simulink model "GoertzelFunction"  (R2014a)
settings: Solver=ode45  StartTime=0.0  StopTime=1  RelTol=1e-3
undefined symbols (not defined in the file): i
libraries: dspsigops x14, dspsrcs4 x7
settings Model: Creator=Tanvir  LastModifiedBy=Tanvir

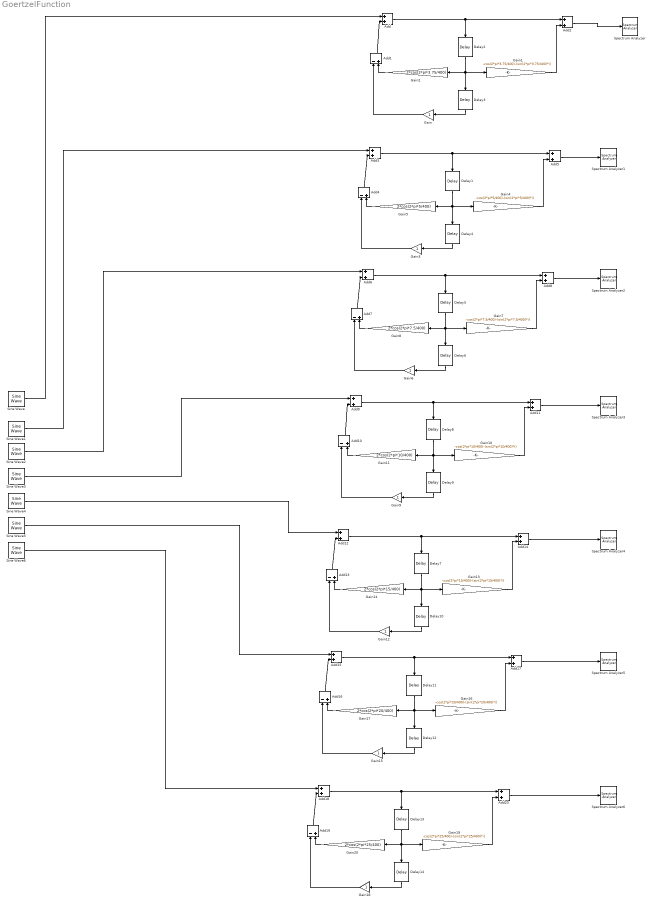
== system GoertzelFunction ==
  Add{,2..3,5..6,8..9,11..12,14..15,17..18,20} (14 alike) : Sum
  Add{1,4,7,10,13,16,19} (7 alike) : Sum  Inputs=-+
  Delay{1..14} (14 alike) : dspsigops/Delay  InputProcessing=Columns as channels (frame based)  dly_unit=Samples  delay=1  ic_detail=off  dif_ic_for_ch=off  dif_ic_for_dly=off  ic=0  reset_popup=None
  Gain{,3,6,9,12,15,18} (7 alike) : Gain
  Gain1 : Gain  Gain=-cos(2*pi*3.75/400)-(sin(2*pi*3.75/400)*i)
  Gain10 : Gain  Gain=-cos(2*pi*10/400)-(sin(2*pi*10/400)*i)
  Gain11 : Gain  Gain=2*cos(2*pi*10/400)
  Gain13 : Gain  Gain=-cos(2*pi*15/400)-(sin(2*pi*15/400)*i)
  Gain14 : Gain  Gain=2*cos(2*pi*15/400)
  Gain16 : Gain  Gain=-cos(2*pi*20/400)-(sin(2*pi*20/400)*i)
  Gain17 : Gain  Gain=2*cos(2*pi*20/400)
  Gain19 : Gain  Gain=-cos(2*pi*25/400)-(sin(2*pi*25/400)*i)
  Gain2 : Gain  Gain=2*cos(2*pi*3.75/400)
  Gain20 : Gain  Gain=2*cos(2*pi*25/400)
  Gain4 : Gain  Gain=-cos(2*pi*5/400)-(sin(2*pi*5/400)*i)
  Gain5 : Gain  Gain=2*cos(2*pi*5/400)
  Gain7 : Gain  Gain=-cos(2*pi*7.5/400)-(sin(2*pi*7.5/400)*i)
  Gain8 : Gain  Gain=2*cos(2*pi*7.5/400)
  Sine Wave : dspsrcs4/Sine Wave  Amplitude=1  Frequency=75  Phase=0  SampleMode=Discrete  OutComplex=Real  CompMethod=Trigonometric fcn  TableSize=Speed  SampleTime=1/8000  SamplesPerFrame=1  ResetState=Restart at time zero  dataType=double  wordLen=16  udDataType=sfix(16)  fracBitsMode=Best precision  numFracBits=15  OutDataTypeStr=double  LastOutDataTypeStr=double
  Sine Wave1 : dspsrcs4/Sine Wave  Amplitude=1  Frequency=100  Phase=0  SampleMode=Discrete  OutComplex=Real  CompMethod=Trigonometric fcn  TableSize=Speed  SampleTime=1/8000  SamplesPerFrame=1  ResetState=Restart at time zero  dataType=double  wordLen=16  udDataType=sfix(16)  fracBitsMode=Best precision  numFracBits=15  OutDataTypeStr=double  LastOutDataTypeStr=double
  Sine Wave2 : dspsrcs4/Sine Wave  Amplitude=1  Frequency=150  Phase=0  SampleMode=Discrete  OutComplex=Real  CompMethod=Trigonometric fcn  TableSize=Speed  SampleTime=1/8000  SamplesPerFrame=1  ResetState=Restart at time zero  dataType=double  wordLen=16  udDataType=sfix(16)  fracBitsMode=Best precision  numFracBits=15  OutDataTypeStr=double  LastOutDataTypeStr=double
  Sine Wave3 : dspsrcs4/Sine Wave  Amplitude=1  Frequency=200  Phase=0  SampleMode=Discrete  OutComplex=Real  CompMethod=Trigonometric fcn  TableSize=Speed  SampleTime=1/8000  SamplesPerFrame=1  ResetState=Restart at time zero  dataType=double  wordLen=16  udDataType=sfix(16)  fracBitsMode=Best precision  numFracBits=15  OutDataTypeStr=double  LastOutDataTypeStr=double
  Sine Wave4 : dspsrcs4/Sine Wave  Amplitude=1  Frequency=300  Phase=0  SampleMode=Discrete  OutComplex=Real  CompMethod=Trigonometric fcn  TableSize=Speed  SampleTime=1/8000  SamplesPerFrame=1  ResetState=Restart at time zero  dataType=double  wordLen=16  udDataType=sfix(16)  fracBitsMode=Best precision  numFracBits=15  OutDataTypeStr=double  LastOutDataTypeStr=double
  Sine Wave5 : dspsrcs4/Sine Wave  Amplitude=1  Frequency=400  Phase=0  SampleMode=Discrete  OutComplex=Real  CompMethod=Trigonometric fcn  TableSize=Speed  SampleTime=1/8000  SamplesPerFrame=1  ResetState=Restart at time zero  dataType=double  wordLen=16  udDataType=sfix(16)  fracBitsMode=Best precision  numFracBits=15  OutDataTypeStr=double  LastOutDataTypeStr=double
  Sine Wave6 : dspsrcs4/Sine Wave  Amplitude=1  Frequency=500  Phase=0  SampleMode=Discrete  OutComplex=Real  CompMethod=Trigonometric fcn  TableSize=Speed  SampleTime=1/8000  SamplesPerFrame=1  ResetState=Restart at time zero  dataType=double  wordLen=16  udDataType=sfix(16)  fracBitsMode=Best precision  numFracBits=15  OutDataTypeStr=double  LastOutDataTypeStr=double
  Spectrum Analyzer{,1..6} (7 alike) : SpectrumAnalyzer
  wires:
  Delay2/1 -> Gain1/1, Gain2/1, Delay3/1
  Delay3/1 -> Gain/1
  Add/1 -> Add2/1, Delay2/1
  Gain/1 -> Add1/1
  Add1/1 -> Add/2
  Gain1/1 -> Add2/2
  Gain2/1 -> Add1/2
  Sine Wave/1 -> Add/1
  Delay1/1 -> Gain4/1, Gain5/1, Delay4/1
  Delay4/1 -> Gain3/1
  Add3/1 -> Add5/1, Delay1/1
  Gain3/1 -> Add4/1
  Add4/1 -> Add3/2
  Gain4/1 -> Add5/2
  Gain5/1 -> Add4/2
  Sine Wave1/1 -> Add3/1
  Delay5/1 -> Gain7/1, Gain8/1, Delay6/1
  Delay6/1 -> Gain6/1
  Add6/1 -> Add8/1, Delay5/1
  Gain6/1 -> Add7/1
  Add7/1 -> Add6/2
  Gain7/1 -> Add8/2
  Gain8/1 -> Add7/2
  Sine Wave2/1 -> Add6/1
  Delay8/1 -> Gain10/1, Gain11/1, Delay9/1
  Delay9/1 -> Gain9/1
  Add9/1 -> Add11/1, Delay8/1
  Gain9/1 -> Add10/1
  Add10/1 -> Add9/2
  Gain10/1 -> Add11/2
  Gain11/1 -> Add10/2
  Sine Wave3/1 -> Add9/1
  Delay7/1 -> Gain13/1, Gain14/1, Delay10/1
  Delay10/1 -> Gain12/1
  Add12/1 -> Add14/1, Delay7/1
  Gain12/1 -> Add13/1
  Add13/1 -> Add12/2
  Gain13/1 -> Add14/2
  Gain14/1 -> Add13/2
  Sine Wave4/1 -> Add12/1
  Delay11/1 -> Gain16/1, Gain17/1, Delay12/1
  Delay12/1 -> Gain15/1
  Add15/1 -> Add17/1, Delay11/1
  Gain15/1 -> Add16/1
  Add16/1 -> Add15/2
  Gain16/1 -> Add17/2
  Gain17/1 -> Add16/2
  Sine Wave5/1 -> Add15/1
  Delay13/1 -> Gain19/1, Gain20/1, Delay14/1
  Delay14/1 -> Gain18/1
  Add18/1 -> Add20/1, Delay13/1
  Gain18/1 -> Add19/1
  Add19/1 -> Add18/2
  Gain19/1 -> Add20/2
  Gain20/1 -> Add19/2
  Sine Wave6/1 -> Add18/1
  Add20/1 -> Spectrum Analyzer6/1
  Add17/1 -> Spectrum Analyzer5/1
  Add14/1 -> Spectrum Analyzer4/1
  Add11/1 -> Spectrum Analyzer3/1
  Add8/1 -> Spectrum Analyzer2/1
  Add5/1 -> Spectrum Analyzer1/1
  Add2/1 -> Spectrum Analyzer/1
